simulink model "Fault"  (R2025b)
settings: configuration reference "code" (kept outside this file)
settings Model: DataDictionary=test.sldd  Creator=rpumpo  LastModifiedBy=rpumpo
settings ConfigSetRef: SourceName=code

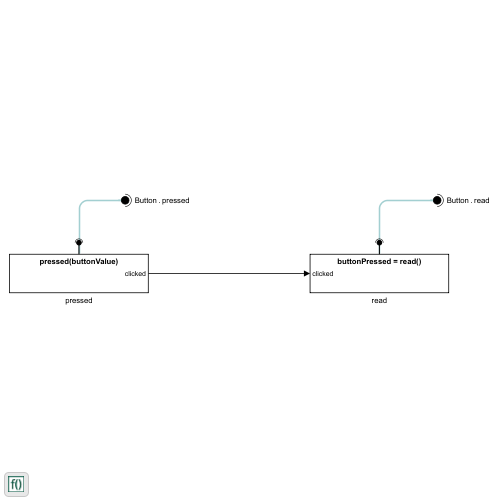
[thumbnail: Simulink's stored preview of the top-level diagram]
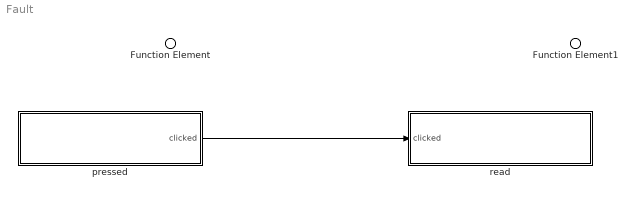
== system Fault ==
  pressed : Subsystem
  read : Subsystem
  Function Element1 : Outport  AllowServiceAccess=on  PortName=Button  Element=read
  Function Element : Outport  AllowServiceAccess=on  PortName=Button  Element=pressed
  wires:
  pressed/1(clicked) -> read/1(clicked)

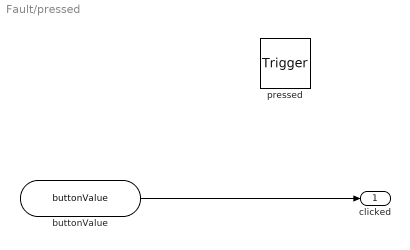
== system Fault/pressed ==
  pressed : TriggerPort  TriggerType=function-call  IsSimulinkFunction=on  FunctionName=pressed  FunctionVisibility=port  ScopeName=Button  VariantControl=(inherit)
  buttonValue : ArgIn  ArgumentName=buttonValue
  clicked : Outport
  wires:
  buttonValue/1 -> clicked/1

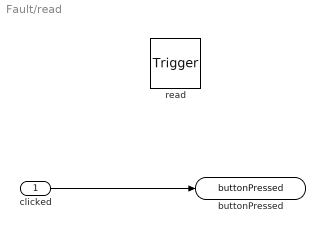
== system Fault/read ==
  clicked : Inport
  read : TriggerPort  TriggerType=function-call  IsSimulinkFunction=on  FunctionName=read  FunctionVisibility=port  ScopeName=Button  VariantControl=(inherit)
  buttonPressed : ArgOut  ArgumentName=buttonPressed
  wires:
  clicked/1 -> buttonPressed/1
